simulink model "sf_aero_guidance_fixpt"  (Simulink 6.0)
settings: Solver=ode45  SolverMode=SingleTasking  StartTime=0.0  StopTime=20  RelTol=1e-3  AbsTol=1e-6
PreLoadFcn:
  | aero_guid_dat
InitFcn:
  | ;
StartFcn:
  | ;
StopFcn:
  | aero_guid_plot;
values from neighbouring files (symbols this model uses):
  g = [0.001016 0.001016 0.001016 0.001016 0.001016 0.001016 0.001016 0.001016 0.0010159999994 0.0010159999994 0.0010159999994 0.0010159999994 ... (38 elements, 38x1)]    [sf_electrohydraulic.mat]
  Ks = 8998.87514061    [sf_electrohydraulic.mat]
undefined symbols (not defined in the file or in its folder): Beamwidth, Cm_el, Cm_q, Cz_el, d2r, d_ref, fin_max, fin_min, h_ini, K_r, l_acc, max_acc, max_gimbal, min_gimbal, pos_tgt, S_ref, theta_tgt, Thrust, tors, v_tgt, wgyro, wn_hom, x_ini
libraries: simulink x11, aerospace x5, fixpt_lib_4 x3
Description:
  | The model represents the dynamics of a missile engaging a target which is flying straight and level.
PreSaveFcn:
  | ;
CloseFcn:
  | h=findobj('type','figure');if ~isempty(h);close(h);end;
settings Model: CovMetricSettings=dcmtr  Creator=The MathWorks Inc.  LastModifiedBy=batserve  ExtModeTrigMode=oneshot  ExtModeArmWhenConnect=off  ExtModeAutoUpdateStatusClock=off  ProdHWDeviceType=Specified
settings DataIOCC: LimitDataPoints=off  SaveOutput=off  StateSaveName=xbase  OutputSaveName=ybase  SignalLoggingName=sigsOut
settings OptimizationCC: BlockReduction=off  BooleanDataType=off
settings DebuggingCC: CheckExecutionContextPreStartOutputMsg=on  CheckExecutionContextRuntimeOutputMsg=on  SolverPrmCheckMsg=none  IntegerOverflowMsg=error  ParameterPrecisionLossMsg=none
settings HardwareCC: ProdBitPerShort=32  ProdBitPerInt=16  ProdHWDeviceType=Specified  TargetUnknown=on

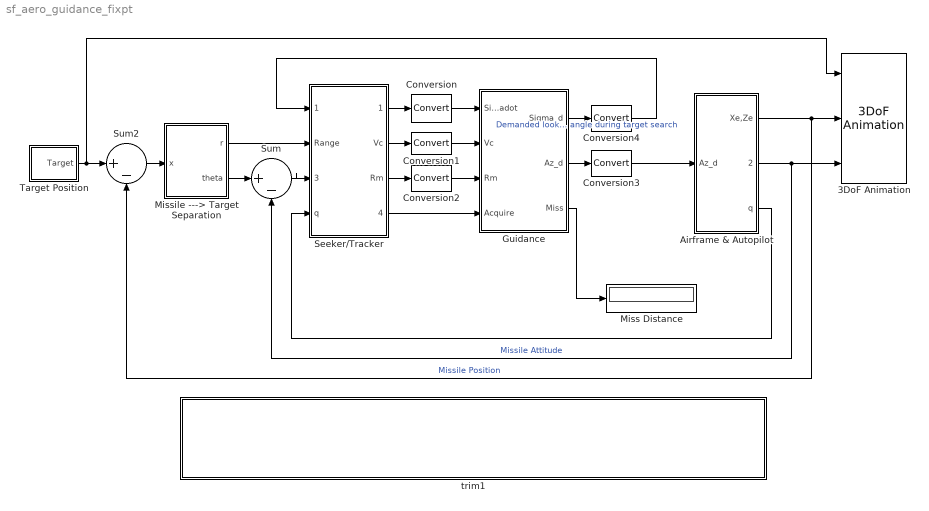
== system sf_aero_guidance_fixpt ==
  3DoF Animation : aerospace/Animation/3DoF Animation  u1=[0 5000 -2000 2000 -5050 -3050]  u2=0.03  u3=1.8  u5=Fly alongside  u6=[200 200 -50]  u7=20  u8=on
  Airframe & Autopilot : Subsystem  PropExecContextAcrossSSBoundary=on
  Conversion : DataTypeConversion  OutDataTypeMode=Specify via dialog  OutScaling=2^-14
  Conversion1 : DataTypeConversion  OutDataTypeMode=Specify via dialog
  Conversion2 : DataTypeConversion  OutScaling=2^-10
  Conversion3 : DataTypeConversion  OutDataTypeMode=Specify via dialog  OutDataType=float('double')  OutScaling=2^-10
  Conversion4 : DataTypeConversion  OutDataTypeMode=Specify via dialog  OutDataType=float('double')  OutScaling=2^-10
  Guidance : Subsystem  PropExecContextAcrossSSBoundary=on
  Miss Distance : Display
  Missile ---> Target Separation : Subsystem  PropExecContextAcrossSSBoundary=on
      mask Type: Cart2Polar
      mask Description:
      | Transformation from cartesian to polar coordinates.
      | [x, y] -> [r, theta]
      | 
      | r = sqrt(x^2 + y^2);
      | theta = atan(y/x);
      mask Help: Unmask this block for more help.
      mask Display: plot(0,0,100,100,[24,20,15,20,20],[85,95,85,95,20],[80,20,95,85,95,85],[70,20,20,15,20,24],[56,56,55,52,50,46],[20,26,31,35,38,42])
  Seeker/Tracker : Subsystem  PropExecContextAcrossSSBoundary=on
  Sum : Sum  Inputs=|+-  SaturateOnIntegerOverflow=on  InputSameDT=on
  Sum2 : Sum  Inputs=|+-  SaturateOnIntegerOverflow=on  InputSameDT=on
  Target Position : Subsystem  PropExecContextAcrossSSBoundary=on
  trim1 : Subsystem  PropExecContextAcrossSSBoundary=on
      settings: AttributesFormatString=\n  OpenFcn=aero_guidance
      mask Display: disp('This model simulates an infrared guidance system using fixed-point math.\n Double-click on this block for the original floating-point version and further details.')
  wires:
  Missile ---> Target Separation/2(theta) -> Sum/1
  Guidance/2(Az_d) -> Conversion3/1
  Seeker/Tracker/2(Vc) -> Conversion1/1
  Seeker/Tracker/3(Rm) -> Conversion2/1
  Guidance/3(Miss) -> Miss Distance/1
  Seeker/Tracker/1(Sigmadot) -> Conversion/1
  Sum/1 -> Seeker/Tracker/3(Look Angle)
  Airframe & Autopilot/3(q) -> Seeker/Tracker/4(q)
  Guidance/1(Sigma_d) -> Conversion4/1  "Demanded look angle during target search"
  Missile ---> Target Separation/1(r) -> Seeker/Tracker/2(Range)
  Airframe & Autopilot/1(Xe,Ze) -> 3DoF Animation/2, Sum2/2  "Missile Position"
  Airframe & Autopilot/2(Attitude) -> 3DoF Animation/3, Sum/2  "Missile Attitude"
  Target Position/1(Target) -> Sum2/1, 3DoF Animation/1
  Sum2/1 -> Missile ---> Target Separation/1(x)
  Seeker/Tracker/4(Acquire) -> Guidance/4(Acquire)
  Conversion/1 -> Guidance/1(Sigmadot)
  Conversion1/1 -> Guidance/2(Vc)
  Conversion2/1 -> Guidance/3(Rm)
  Conversion3/1 -> Airframe & Autopilot/1(Az_d)
  Conversion4/1 -> Seeker/Tracker/1(Sigma_d)

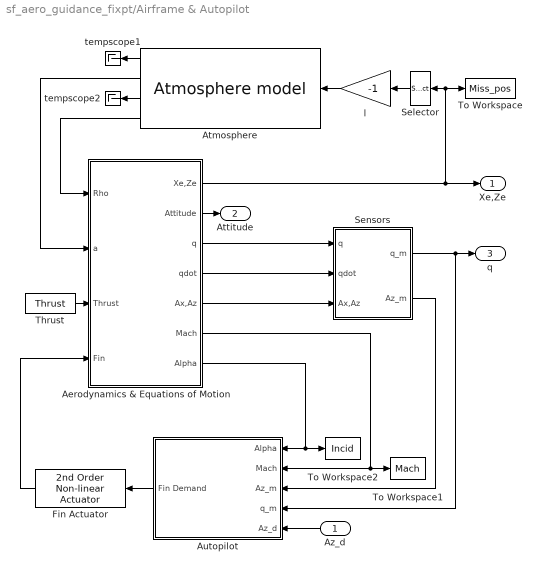
== system sf_aero_guidance_fixpt/Airframe & Autopilot ==
  Az_d : Inport  Orientation=left  Port=1  SampleTime=0  LatchInput=off
  Aerodynamics & Equations of Motion : Subsystem  PropExecContextAcrossSSBoundary=on
  Atmosphere : aerospace/Atmosphere/Atmosphere model  Orientation=left
  Autopilot : Subsystem  Orientation=left  PropExecContextAcrossSSBoundary=on
  Fin Actuator : aerospace/Actuators/2nd Order Non-linear Actuator  Orientation=left  wn_fin=wn_fin  z_fin=z_fin  fin_max=fin_max  fin_min=fin_min  fin_maxrate=fin_maxrate  fin_act_0=fin_act_0
  Selector : Selector  Orientation=left  Elements=[2]  InputPortWidth=2
  Sensors : Subsystem  PropExecContextAcrossSSBoundary=on
  Thrust : Constant  Value=Thrust
  To Workspace : ToWorkspace  VariableName=Miss_pos  SampleTime=-1  SaveFormat=Structure With Time
  To Workspace1 : ToWorkspace  VariableName=Mach  SampleTime=-1  SaveFormat=Structure With Time
  To Workspace2 : ToWorkspace  VariableName=Incid  SampleTime=-1  SaveFormat=Structure With Time
  l : Gain  Orientation=left  Gain=-1  SaturateOnIntegerOverflow=on
  tempscope1 : Terminator
  tempscope2 : Terminator
  Xe,Ze : Outport  InitialOutput=0
  Attitude : Outport  Port=2  InitialOutput=0
  q : Outport  Port=3  InitialOutput=0
  wires:
  Aerodynamics & Equations of Motion/2(Attitude) -> Attitude/1
  Thrust/1 -> Aerodynamics & Equations of Motion/3(Thrust)
  Atmosphere/3 -> tempscope2/1
  Atmosphere/4 -> Aerodynamics & Equations of Motion/1(Rho)
  Atmosphere/1 -> tempscope1/1
  Atmosphere/2 -> Aerodynamics & Equations of Motion/2(a)
  Selector/1 -> l/1
  l/1 -> Atmosphere/1
  Aerodynamics & Equations of Motion/5(Ax,Az) -> Sensors/3(Ax,Az)
  Aerodynamics & Equations of Motion/4(qdot) -> Sensors/2(qdot)
  Aerodynamics & Equations of Motion/1(Xe,Ze) -> Xe,Ze/1, To Workspace/1, Selector/1
  Az_d/1 -> Autopilot/5(Az_d)
  Autopilot/1(Fin Demand) -> Fin Actuator/1
  Fin Actuator/1 -> Aerodynamics & Equations of Motion/4(Fin)
  Aerodynamics & Equations of Motion/7(Alpha) -> Autopilot/1(Alpha), To Workspace2/1
  Sensors/2(Az_m) -> Autopilot/3(Az_m)
  Aerodynamics & Equations of Motion/6(Mach) -> Autopilot/2(Mach), To Workspace1/1
  Sensors/1(q_m) -> Autopilot/4(q_m), q/1
  Aerodynamics & Equations of Motion/3(q) -> Sensors/1(q)

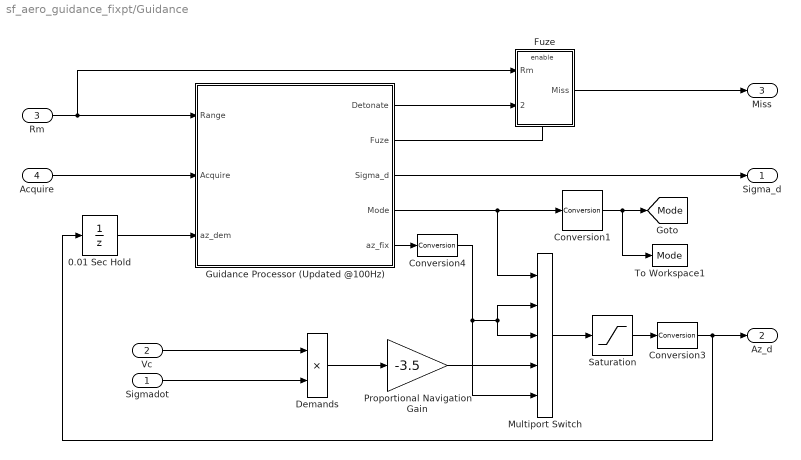
== system sf_aero_guidance_fixpt/Guidance ==
  Sigmadot : Inport  Port=1  SampleTime=0.01  LatchInput=off
  Vc : Inport  Port=2  SampleTime=0.01  LatchInput=off
  Rm : Inport  Port=3  SampleTime=0.01  LatchInput=off
  Acquire : Inport  Port=4  SampleTime=0.01  LatchInput=off
  0.01 Sec Hold : UnitDelay  SampleTime=0.01
  Conversion1 : fixpt_lib_4/Data Type/Conversion  ConvertRealWorld=Real World Value  OutputDataTypeScalingMode=Specify via dialog  OutDataType=float('double')  OutScaling=2^-10  DoSatur=off
  Conversion3 : fixpt_lib_4/Data Type/Conversion  ConvertRealWorld=Real World Value  OutDataType=float('double')  OutScaling=2^-10  DoSatur=off
  Conversion4 : fixpt_lib_4/Data Type/Conversion  ConvertRealWorld=Real World Value  OutDataType=float('double')  OutScaling=2^-10  DoSatur=off
  Demands : Product  OutDataTypeMode=Specify via dialog  OutScaling=2^-6  SaturateOnIntegerOverflow=on
  Fuze : Subsystem  TreatAsAtomicUnit=on  PropExecContextAcrossSSBoundary=on
  Guidance Processor (Updated @100Hz) : Stateflow chart  PropExecContextAcrossSSBoundary=on
  Multiport Switch : MultiPortSwitch  InputSameDT=on
  Proportional Navigation Gain : Gain  Gain=-3.5  SaturateOnIntegerOverflow=on
  Saturation : Saturate  UpperLimit=max_acc  LowerLimit=-max_acc
  To Workspace1 : ToWorkspace  VariableName=Mode  SaveFormat=Structure With Time
  Sigma_d : Outport
  Az_d : Outport  Port=2
  Miss : Outport  Port=3
  tag scope: Mode=global
  wires:
  Fuze/1("Miss ") -> Miss/1
  Rm/1 -> Guidance Processor (Updated @100Hz)/1(Range), Fuze/1(Rm)
  Guidance Processor (Updated @100Hz)/4(Mode) -> Multiport Switch/1, Conversion1/1
  Acquire/1 -> Guidance Processor (Updated @100Hz)/2(Acquire)
  Multiport Switch/1 -> Saturation/1
  Saturation/1 -> Conversion3/1
  Guidance Processor (Updated @100Hz)/5(az_fix) -> Conversion4/1
  0.01 Sec Hold/1 -> Guidance Processor (Updated @100Hz)/3(az_dem)
  Guidance Processor (Updated @100Hz)/2(Fuze) -> Fuze/Enable
  Sigmadot/1 -> Demands/2
  Proportional Navigation Gain/1 -> Multiport Switch/4
  Vc/1 -> Demands/1
  Demands/1 -> Proportional Navigation Gain/1
  Guidance Processor (Updated @100Hz)/3(Sigma_d) -> Sigma_d/1
  Conversion1/1 -> [Mode], To Workspace1/1
  Guidance Processor (Updated @100Hz)/1(Detonate) -> Fuze/2(Detonate)
  Conversion3/1 -> Az_d/1, 0.01 Sec Hold/1
  Conversion4/1 -> Multiport Switch/2, Multiport Switch/3, Multiport Switch/5

== system sf_aero_guidance_fixpt/Missile ---> Target Separation ==
  x : Inport  Port=1  LatchInput=off
  Range : Fcn  Expr=hypot(u[1],u[2])
  Sightline Angle : Fcn  Expr=atan2(-u[2],u[1])
  r : Outport  InitialOutput=0
  theta : Outport  Port=2  InitialOutput=0
  wires:
  x/1 -> Sightline Angle/1, Range/1
  Range/1 -> r/1
  Sightline Angle/1 -> theta/1

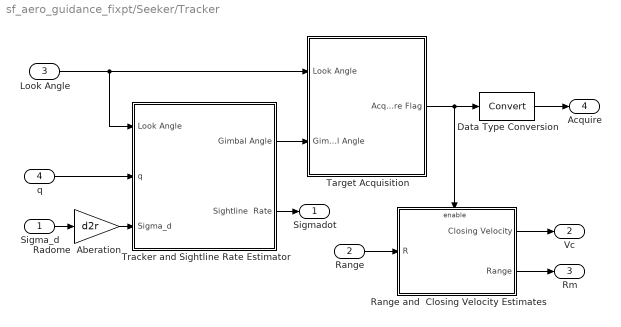
== system sf_aero_guidance_fixpt/Seeker/Tracker ==
  Sigma_d : Inport  Port=1  LatchInput=off
  Range : Inport  Port=2  LatchInput=off
  Look Angle : Inport  Port=3  LatchInput=off
  q : Inport  Port=4  LatchInput=off
  Data Type Conversion : DataTypeConversion  OutDataTypeMode=boolean  SaturateOnIntegerOverflow=on  RndMeth=Zero
  Radome  Aberation : Gain  Gain=d2r  SaturateOnIntegerOverflow=on
  Range and  Closing Velocity Estimates : Subsystem  TreatAsAtomicUnit=on  PropExecContextAcrossSSBoundary=on
  Target Acquisition : Subsystem  PropExecContextAcrossSSBoundary=on
  Tracker and Sightline Rate Estimator : Subsystem  PropExecContextAcrossSSBoundary=on
  Sigmadot : Outport
  Vc : Outport  Port=2
  Rm : Outport  Port=3
  Acquire : Outport  Port=4
  wires:
  Tracker and Sightline Rate Estimator/2(Sightline  Rate) -> Sigmadot/1
  Radome  Aberation/1 -> Tracker and Sightline Rate Estimator/3(Sigma_d)
  Tracker and Sightline Rate Estimator/1("Gimbal Angle ") -> Target Acquisition/2(Gimbal Angle)
  Target Acquisition/1(Acquire Flag) -> Range and  Closing Velocity Estimates/Enable, Data Type Conversion/1
  q/1 -> Tracker and Sightline Rate Estimator/2(q)
  Look Angle/1 -> Target Acquisition/1(Look Angle), Tracker and Sightline Rate Estimator/1(Look Angle)
  Range/1 -> Range and  Closing Velocity Estimates/1(R)
  Range and  Closing Velocity Estimates/2(Range) -> Rm/1
  Range and  Closing Velocity Estimates/1(Closing Velocity) -> Vc/1
  Sigma_d/1 -> Radome  Aberation/1
  Data Type Conversion/1 -> Acquire/1

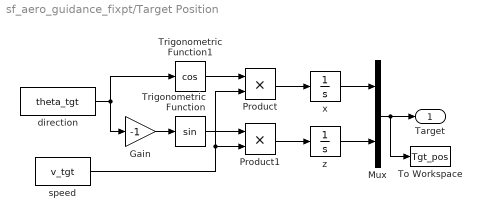
== system sf_aero_guidance_fixpt/Target Position ==
  Gain : Gain  Gain=-1  SaturateOnIntegerOverflow=on
  Mux : Mux  Inputs=2
  Product : Product  SaturateOnIntegerOverflow=on  InputSameDT=on
  Product1 : Product  SaturateOnIntegerOverflow=on  InputSameDT=on
  To Workspace : ToWorkspace  VariableName=Tgt_pos  SampleTime=-1  SaveFormat=Structure
  Trigonometric Function : Trigonometry
  Trigonometric Function1 : Trigonometry  Operator=cos
  direction : Constant  Value=theta_tgt
  speed : Constant  Value=v_tgt
  x : Integrator  InitialCondition=pos_tgt(1)  ZeroCross=off
  z : Integrator  InitialCondition=pos_tgt(2)  ZeroCross=off
  Target : Outport
  wires:
  x/1 -> Mux/1
  z/1 -> Mux/2
  Product/1 -> x/1
  Product1/1 -> z/1
  speed/1 -> Product/2, Product1/2
  Trigonometric Function/1 -> Product1/1
  Trigonometric Function1/1 -> Product/1
  direction/1 -> Trigonometric Function1/1, Gain/1
  Gain/1 -> Trigonometric Function/1
  Mux/1 -> Target/1, To Workspace/1

== system sf_aero_guidance_fixpt/trim1 ==

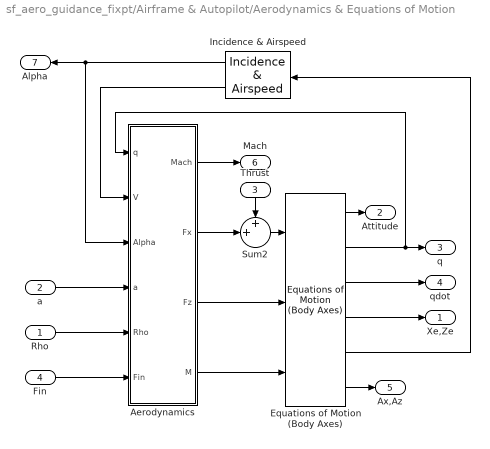
== system sf_aero_guidance_fixpt/Airframe & Autopilot/Aerodynamics & Equations of Motion ==
  Rho : Inport  Port=1  LatchInput=off
  a : Inport  Port=2  LatchInput=off
  Thrust : Inport  Orientation=down  Port=3  LatchInput=off
  Fin : Inport  Port=4  LatchInput=off
  " Equations of Motion (Body Axes)" : aerospace/3DoF Equations of Motion / Equations of Motion (Body Axes)  v_ini=v_ini  theta_ini=theta_ini  alpha_ini=alpha_ini  q_ini=q_ini  pos_ini=[x_ini -h_ini]  mass=mass  Iyy=Iyy  g=g
  Aerodynamics : Subsystem  PropExecContextAcrossSSBoundary=on
  Incidence & Airspeed : aerospace/3DoF Equations of Motion /Incidence  & Airspeed  Orientation=left
  Sum2 : Sum  Inputs=++|  SaturateOnIntegerOverflow=on  InputSameDT=on
  Xe,Ze : Outport  InitialOutput=0
  Attitude : Outport  Port=2  InitialOutput=0
  q : Outport  Port=3  InitialOutput=0
  qdot : Outport  Port=4  InitialOutput=0
  Ax,Az : Outport  Port=5  InitialOutput=0
  Mach : Outport  Port=6  InitialOutput=0
  Alpha : Outport  Orientation=left  Port=7  InitialOutput=0
  wires:
  Aerodynamics/1(" Mach") -> Mach/1
  Aerodynamics/4(" M") -> " Equations of Motion (Body Axes)"/3
  Sum2/1 -> " Equations of Motion (Body Axes)"/1
  Incidence & Airspeed/1 -> Aerodynamics/3(Alpha), Alpha/1
  Rho/1 -> Aerodynamics/5(Rho)
  a/1 -> Aerodynamics/4(a)
  Fin/1 -> Aerodynamics/6(Fin)
  Incidence & Airspeed/2 -> Aerodynamics/2(V)
  Aerodynamics/3(Fz) -> " Equations of Motion (Body Axes)"/2
  Aerodynamics/2(Fx) -> Sum2/2
  Thrust/1 -> Sum2/1
  " Equations of Motion (Body Axes)"/2 -> q/1, Aerodynamics/1(q)
  " Equations of Motion (Body Axes)"/3 -> qdot/1
  " Equations of Motion (Body Axes)"/1 -> Attitude/1
  " Equations of Motion (Body Axes)"/4 -> Xe,Ze/1
  " Equations of Motion (Body Axes)"/6 -> Ax,Az/1
  " Equations of Motion (Body Axes)"/5 -> Incidence & Airspeed/1

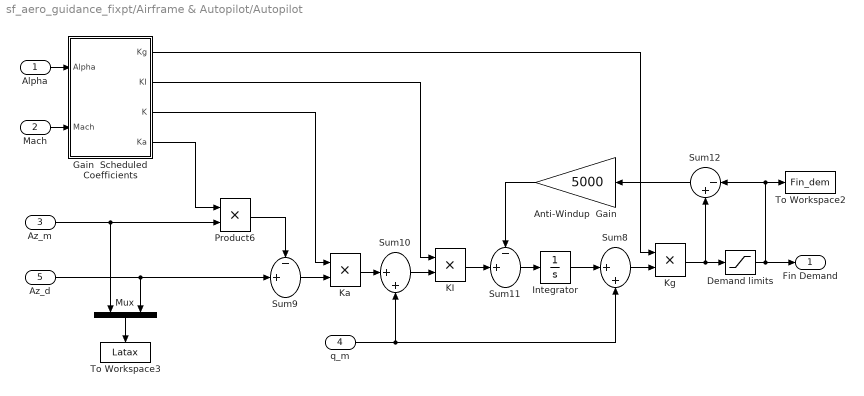
== system sf_aero_guidance_fixpt/Airframe & Autopilot/Autopilot ==
  Alpha : Inport  Port=1  LatchInput=off
  Mach : Inport  Port=2  LatchInput=off
  Az_m : Inport  Port=3  LatchInput=off
  q_m : Inport  Port=4  LatchInput=off
  Az_d : Inport  Port=5  LatchInput=off
  Anti-Windup  Gain : Gain  Orientation=left  Gain=5000  SaturateOnIntegerOverflow=on
  "Demand limits " : Saturate  UpperLimit=fin_max  LowerLimit=fin_min  ZeroCross=off
  Gain  Scheduled Coefficients : Subsystem  PropExecContextAcrossSSBoundary=on
  Integrator : Integrator  ZeroCross=off
  KI : Product  SaturateOnIntegerOverflow=on  InputSameDT=on
  Ka : Product  SaturateOnIntegerOverflow=on  InputSameDT=on
  Kg : Product  SaturateOnIntegerOverflow=on  InputSameDT=on
  Mux : Mux  Orientation=down  Inputs=2
  Product6 : Product  SaturateOnIntegerOverflow=on  InputSameDT=on
  Sum10 : Sum  Inputs=|++  SaturateOnIntegerOverflow=on  InputSameDT=on
  Sum11 : Sum  Inputs=-+|  SaturateOnIntegerOverflow=on  InputSameDT=on
  Sum12 : Sum  Orientation=left  Inputs=|-+  SaturateOnIntegerOverflow=on  InputSameDT=on
  Sum8 : Sum  Inputs=|++  SaturateOnIntegerOverflow=on  InputSameDT=on
  Sum9 : Sum  Inputs=-+|  SaturateOnIntegerOverflow=on  InputSameDT=on
  To Workspace2 : ToWorkspace  VariableName=Fin_dem  SampleTime=-1  SaveFormat=Structure With Time
  To Workspace3 : ToWorkspace  VariableName=Latax  SampleTime=-1  SaveFormat=Structure With Time
      settings: Orientation=down
  Fin Demand : Outport  InitialOutput=0
  wires:
  Mach/1 -> Gain  Scheduled Coefficients/2(Mach)
  Alpha/1 -> Gain  Scheduled Coefficients/1(Alpha)
  Kg/1 -> Sum12/2, "Demand limits "/1
  Gain  Scheduled Coefficients/1("Kg ") -> Kg/1
  Gain  Scheduled Coefficients/3("K ") -> Ka/1
  Gain  Scheduled Coefficients/2("KI ") -> KI/1
  Anti-Windup  Gain/1 -> Sum11/1
  Sum8/1 -> Kg/2
  Integrator/1 -> Sum8/1
  Sum11/1 -> Integrator/1
  Product6/1 -> Sum9/1
  Sum9/1 -> Ka/2
  Ka/1 -> Sum10/1
  Sum10/1 -> KI/2
  KI/1 -> Sum11/2
  Sum12/1 -> Anti-Windup  Gain/1
  Az_d/1 -> Mux/2, Sum9/2
  Mux/1 -> To Workspace3/1
  q_m/1 -> Sum10/2, Sum8/2
  "Demand limits "/1 -> Fin Demand/1, Sum12/1, To Workspace2/1
  Az_m/1 -> Mux/1, Product6/2
  Gain  Scheduled Coefficients/4("Ka ") -> Product6/1

== system sf_aero_guidance_fixpt/Airframe & Autopilot/Sensors ==
  q : Inport  Port=1  LatchInput=off
  qdot : Inport  Port=2  LatchInput=off
  Ax,Az : Inport  Port=3  LatchInput=off
  Selector : Selector  Elements=[2]  InputPortWidth=2
  Sum : Sum  Inputs=-+|  SaturateOnIntegerOverflow=on  InputSameDT=on
  l : Gain  Gain=l_acc  SaturateOnIntegerOverflow=on
  q_m : Outport  InitialOutput=0
  Az_m : Outport  Port=2  InitialOutput=0
  wires:
  Selector/1 -> Sum/2
  Ax,Az/1 -> Selector/1
  q/1 -> q_m/1  "Rate Gyro"
  l/1 -> Sum/1
  Sum/1 -> Az_m/1  "Accelerometer"
  qdot/1 -> l/1

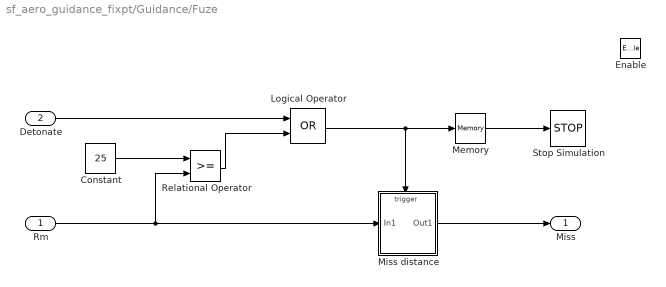
== system sf_aero_guidance_fixpt/Guidance/Fuze ==
  Rm : Inport  Port=1  LatchInput=off
  Detonate : Inport  Port=2  LatchInput=off
  Enable : EnablePort  ZeroCross=off
  Constant : Constant  Value=25
  Logical Operator : Logic  Operator=OR
  Memory : Memory  InheritSampleTime=on
  Miss distance : Subsystem  TreatAsAtomicUnit=on  PropExecContextAcrossSSBoundary=on
  Relational Operator : RelationalOperator  LogicOutDataTypeMode=Boolean
  Stop Simulation : Stop
  "Miss " : Outport
  wires:
  Detonate/1 -> Logical Operator/1
  Rm/1 -> Miss distance/1(In1), Relational Operator/2
  Relational Operator/1 -> Logical Operator/2
  Memory/1 -> Stop Simulation/1
  Miss distance/1(Out1) -> "Miss "/1
  Logical Operator/1 -> Miss distance/Trigger, Memory/1
  Constant/1 -> Relational Operator/1

== system sf_aero_guidance_fixpt/Seeker/Tracker/Range and  Closing Velocity Estimates ==
  R : Inport  Port=1  LatchInput=off
  Enable : EnablePort  Orientation=left  StatesWhenEnabling=reset  ZeroCross=off
  Bandwidth of Estimator : Gain  Gain=wn_hom  SaturateOnIntegerOverflow=on
  Initialized at acquisition : Integrator  Orientation=left  InitialConditionSource=external  ZeroCross=off
  Rdot ---> Vc : Gain  Gain=-1  SaturateOnIntegerOverflow=on
  Sum : Sum  Inputs=|+-  SaturateOnIntegerOverflow=on  InputSameDT=on
  Closing Velocity : Outport  InitialOutput=0
  Range : Outport  Port=2  InitialOutput=0
  wires:
  R/1 -> Range/1, Initialized at acquisition/2, Sum/1
  Sum/1 -> Bandwidth of Estimator/1
  Initialized at acquisition/1 -> Sum/2
  Bandwidth of Estimator/1 -> Rdot ---> Vc/1, Initialized at acquisition/1
  Rdot ---> Vc/1 -> Closing Velocity/1

== system sf_aero_guidance_fixpt/Seeker/Tracker/Target Acquisition ==
  Look Angle : Inport  Port=1  LatchInput=off
  Gimbal Angle : Inport  Port=2  LatchInput=off
  Abs : Abs  SaturateOnIntegerOverflow=on
  Beamwidth : Constant  Value=Beamwidth/2
  Mux : Mux  Inputs=2
  Relational Operator : RelationalOperator  Operator=<  InputSameDT=on
  Sum : Sum  Inputs=+-  SaturateOnIntegerOverflow=on  InputSameDT=on
  To Workspace2 : ToWorkspace  VariableName=Gimbal  SampleTime=-1  SaveFormat=Structure With Time
  Acquire Flag : Outport
  wires:
  Look Angle/1 -> Sum/2, Mux/2
  Gimbal Angle/1 -> Sum/1, Mux/1
  Mux/1 -> To Workspace2/1
  Sum/1 -> Abs/1
  Beamwidth/1 -> Relational Operator/2
  Relational Operator/1 -> Acquire Flag/1
  Abs/1 -> Relational Operator/1

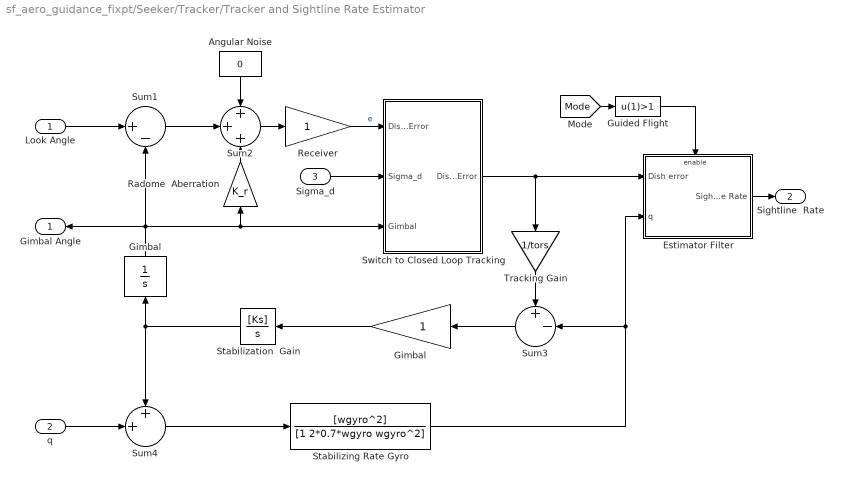
== system sf_aero_guidance_fixpt/Seeker/Tracker/Tracker and Sightline Rate Estimator ==
  Look Angle : Inport  Port=1  LatchInput=off
  q : Inport  Port=2  LatchInput=off
  Sigma_d : Inport  Port=3  LatchInput=off
  Angular Noise : Constant  Orientation=down  Value=0
  Estimator Filter : Subsystem  TreatAsAtomicUnit=on  PropExecContextAcrossSSBoundary=on
  Gimbal : Gain  Orientation=left  SaturateOnIntegerOverflow=on
  "Gimbal " : Integrator  Orientation=up  LimitOutput=on  UpperSaturationLimit=max_gimbal  LowerSaturationLimit=min_gimbal  ZeroCross=off
  Guided Flight : Fcn  Expr=u(1)>1
  Radome  Aberration : Gain  Orientation=up  Gain=K_r  SaturateOnIntegerOverflow=on
  Receiver : Gain  SaturateOnIntegerOverflow=on
  Stabilization  Gain : TransferFcn  Orientation=left  Numerator=[Ks]  Denominator=[1 0]
  Stabilizing Rate Gyro : TransferFcn  Numerator=[wgyro^2]  Denominator=[1 2*0.7*wgyro wgyro^2]
  Sum1 : Sum  Inputs=|+-  SaturateOnIntegerOverflow=on  InputSameDT=on
  Sum2 : Sum  Inputs=+++  SaturateOnIntegerOverflow=on  InputSameDT=on
  Sum3 : Sum  Orientation=left  Inputs=+-|  SaturateOnIntegerOverflow=on  InputSameDT=on
  Sum4 : Sum  Inputs=++|  SaturateOnIntegerOverflow=on  InputSameDT=on
  Switch to Closed Loop Tracking : Subsystem  PropExecContextAcrossSSBoundary=on
  Tracking Gain : Gain  Orientation=down  Gain=1/tors  SaturateOnIntegerOverflow=on
  "Gimbal Angle " : Outport  Orientation=left
  Sightline  Rate : Outport  Port=2
  wires:
  "Gimbal "/1 -> Sum1/2, Radome  Aberration/1, Switch to Closed Loop Tracking/3(Gimbal), "Gimbal Angle "/1
  Stabilization  Gain/1 -> "Gimbal "/1, Sum4/1
  Gimbal/1 -> Stabilization  Gain/1
  Look Angle/1 -> Sum1/1
  Sum2/1 -> Receiver/1
  Receiver/1 -> Switch to Closed Loop Tracking/1(Dish Error)  "e"
  Sigma_d/1 -> Switch to Closed Loop Tracking/2(Sigma_d)
  Estimator Filter/1(Sightline Rate) -> Sightline  Rate/1
  Radome  Aberration/1 -> Sum2/3
  Sum1/1 -> Sum2/2
  Angular Noise/1 -> Sum2/1
  Sum4/1 -> Stabilizing Rate Gyro/1
  q/1 -> Sum4/2
  Stabilizing Rate Gyro/1 -> Sum3/2, Estimator Filter/2(q)
  Sum3/1 -> Gimbal/1
  Tracking Gain/1 -> Sum3/1
  Switch to Closed Loop Tracking/1(Dish Error) -> Tracking Gain/1, Estimator Filter/1(Dish error)
  Guided Flight/1 -> Estimator Filter/Enable
  [Mode] -> Guided Flight/1

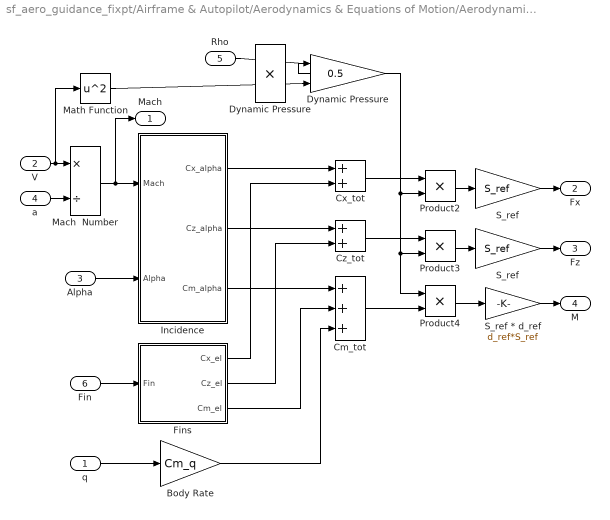
== system sf_aero_guidance_fixpt/Airframe & Autopilot/Aerodynamics & Equations of Motion/Aerodynamics ==
  q : Inport  Port=1  LatchInput=off
  V : Inport  Port=2  LatchInput=off
  Alpha : Inport  Port=3  LatchInput=off
  a : Inport  Port=4  LatchInput=off
  Rho : Inport  Port=5  LatchInput=off
  Fin : Inport  Port=6  LatchInput=off
  Body Rate : Gain  Gain=Cm_q  SaturateOnIntegerOverflow=on
  Cm_tot : Sum  Inputs=+++  SaturateOnIntegerOverflow=on  InputSameDT=on
  Cx_tot : Sum  SaturateOnIntegerOverflow=on  InputSameDT=on
  Cz_tot : Sum  SaturateOnIntegerOverflow=on  InputSameDT=on
  Dynamic Pressure : Gain  Gain=0.5  SaturateOnIntegerOverflow=on
  Dynamic Pressure : Product  SaturateOnIntegerOverflow=on  InputSameDT=on
  Fins : Subsystem  PropExecContextAcrossSSBoundary=on
  Incidence : Subsystem  PropExecContextAcrossSSBoundary=on
  Mach  Number : Product  Inputs=*/  SaturateOnIntegerOverflow=on  InputSameDT=on
  Math Function : Math  Operator=square  SaturateOnIntegerOverflow=on
  Product2 : Product  SaturateOnIntegerOverflow=on  InputSameDT=on
  Product3 : Product  SaturateOnIntegerOverflow=on  InputSameDT=on
  Product4 : Product  SaturateOnIntegerOverflow=on  InputSameDT=on
  S_ref : Gain  Gain=S_ref  SaturateOnIntegerOverflow=on
  S_ref * d_ref : Gain  Gain=d_ref*S_ref  SaturateOnIntegerOverflow=on
  "S_ref " : Gain  Gain=S_ref  SaturateOnIntegerOverflow=on
  " Mach" : Outport  InitialOutput=0
  Fx : Outport  Port=2  InitialOutput=[0]
  Fz : Outport  Port=3  InitialOutput=0
  " M" : Outport  Port=4  InitialOutput=0
  wires:
  Math Function/1 -> Dynamic Pressure/2
  Rho/1 -> Dynamic Pressure/1
  Dynamic Pressure/1 -> Dynamic Pressure/1
  Dynamic Pressure/1 -> Product2/2, Product3/2, Product4/1
  V/1 -> Math Function/1, Mach  Number/1
  Incidence/1(Cx_alpha) -> Cx_tot/1
  Fins/1(Cx_el) -> Cx_tot/2
  Incidence/2(Cz_alpha) -> Cz_tot/1
  Fins/2(Cz_el) -> Cz_tot/2
  Incidence/3(Cm_alpha) -> Cm_tot/1
  Fins/3(Cm_el) -> Cm_tot/2
  Body Rate/1 -> Cm_tot/3
  a/1 -> Mach  Number/2
  Alpha/1 -> Incidence/2(Alpha)
  Cx_tot/1 -> Product2/1
  Cz_tot/1 -> Product3/1
  Product2/1 -> S_ref/1
  S_ref/1 -> Fx/1
  Product3/1 -> "S_ref "/1
  "S_ref "/1 -> Fz/1
  Fin/1 -> Fins/1(Fin)
  S_ref * d_ref/1 -> " M"/1
  Product4/1 -> S_ref * d_ref/1
  Cm_tot/1 -> Product4/2
  q/1 -> Body Rate/1
  Mach  Number/1 -> " Mach"/1, Incidence/1(Mach)

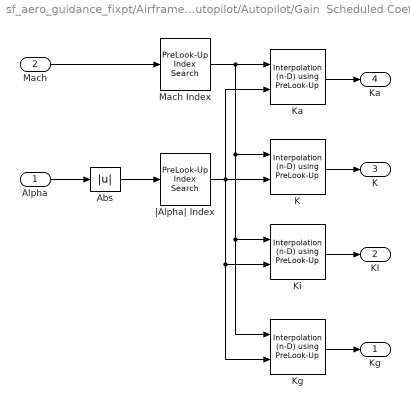
== system sf_aero_guidance_fixpt/Airframe & Autopilot/Autopilot/Gain  Scheduled Coefficients ==
  Alpha : Inport  Port=1  LatchInput=off
  Mach : Inport  Port=2  LatchInput=off
  Abs : Abs  SaturateOnIntegerOverflow=on
  K : simulink/Look-Up Tables/Interpolation (n-D) using PreLook-Up  numDimsPopupSelect=2  explicitNumDims=2  table=K  interpMethod=Linear  extrapMethod=Linear  rangeErrorMode=None
  Ka : simulink/Look-Up Tables/Interpolation (n-D) using PreLook-Up  numDimsPopupSelect=2  explicitNumDims=2  table=Ka  interpMethod=Linear  extrapMethod=Linear  rangeErrorMode=None
  Kg : simulink/Look-Up Tables/Interpolation (n-D) using PreLook-Up  numDimsPopupSelect=2  explicitNumDims=2  table=Kg  interpMethod=Linear  extrapMethod=Linear  rangeErrorMode=None
  Ki : simulink/Look-Up Tables/Interpolation (n-D) using PreLook-Up  numDimsPopupSelect=2  explicitNumDims=2  table=Ki  interpMethod=Linear  extrapMethod=Linear  rangeErrorMode=None
  Mach Index : simulink/Look-Up Tables/PreLook-Up Index Search  bpData=M_sch  searchMode=Binary Search  cacheBpFlag=on  outputFlag=off  extrapMode=Linear Extrapolation  rangeErrorMode=None
  |Alpha| Index : simulink/Look-Up Tables/PreLook-Up Index Search  bpData=alpha_sch  searchMode=Binary Search  cacheBpFlag=on  outputFlag=off  extrapMode=Linear Extrapolation  rangeErrorMode=None
  "Kg " : Outport  InitialOutput=0
  "KI " : Outport  Port=2  InitialOutput=0
  "K " : Outport  Port=3  InitialOutput=0
  "Ka " : Outport  Port=4  InitialOutput=0
  wires:
  Alpha/1 -> Abs/1
  Mach Index/1 -> Ka/1, K/1, Ki/1, Kg/1
  |Alpha| Index/1 -> Ka/2, K/2, Ki/2, Kg/2
  Ka/1 -> "Ka "/1
  K/1 -> "K "/1
  Ki/1 -> "KI "/1
  Kg/1 -> "Kg "/1
  Abs/1 -> |Alpha| Index/1
  Mach/1 -> Mach Index/1

== system sf_aero_guidance_fixpt/Guidance/Fuze/Miss distance ==
  In1 : Inport  Port=1  LatchInput=off
  Trigger : TriggerPort
  Out1 : Outport
  wires:
  In1/1 -> Out1/1

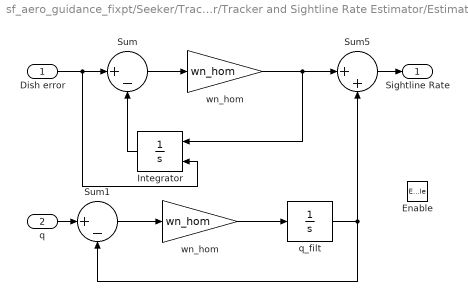
== system sf_aero_guidance_fixpt/Seeker/Tracker/Tracker and Sightline Rate Estimator/Estimator Filter ==
  Dish error : Inport  Port=1  LatchInput=off
  q : Inport  Port=2  LatchInput=off
  Enable : EnablePort  StatesWhenEnabling=reset  ZeroCross=off
  Integrator : Integrator  Orientation=left  InitialConditionSource=external  ZeroCross=off
  Sum : Sum  Inputs=|+-  SaturateOnIntegerOverflow=on  InputSameDT=on
  Sum1 : Sum  Inputs=|+-  SaturateOnIntegerOverflow=on  InputSameDT=on
  Sum5 : Sum  Inputs=|++  SaturateOnIntegerOverflow=on  InputSameDT=on
  q_filt : Integrator  ZeroCross=off
  wn_hom : Gain  Gain=wn_hom  SaturateOnIntegerOverflow=on
  "wn_hom  " : Gain  Gain=wn_hom  SaturateOnIntegerOverflow=on
  Sightline Rate : Outport  InitialOutput=0
  wires:
  Dish error/1 -> Sum/1, Integrator/2
  Sum/1 -> wn_hom/1
  Integrator/1 -> Sum/2
  Sum5/1 -> Sightline Rate/1
  wn_hom/1 -> Integrator/1, Sum5/1
  q/1 -> Sum1/1
  Sum1/1 -> "wn_hom  "/1
  "wn_hom  "/1 -> q_filt/1
  q_filt/1 -> Sum5/2, Sum1/2

== system sf_aero_guidance_fixpt/Seeker/Tracker/Tracker and Sightline Rate Estimator/Switch to Closed Loop Tracking ==
  Dish Error : Inport  Port=1  LatchInput=off
  Sigma_d : Inport  Port=2  LatchInput=off
  Gimbal : Inport  Port=3  LatchInput=off
  Guided Flight : Fcn  Expr=u(1)>1
  Sum5 : Sum  Inputs=-+  SaturateOnIntegerOverflow=on  InputSameDT=on
  Switch2 : Switch  Threshold=0.5  InputSameDT=on
  Dish Error : Outport
  wires:
  [Mode] -> Guided Flight/1
  Guided Flight/1 -> Switch2/2
  Sum5/1 -> Switch2/3
  Dish Error/1 -> Switch2/1
  Switch2/1 -> Dish Error/1
  Sigma_d/1 -> Sum5/2
  Gimbal/1 -> Sum5/1

== system sf_aero_guidance_fixpt/Airframe & Autopilot/Aerodynamics & Equations of Motion/Aerodynamics/Fins ==
  Fin : Inport  Port=1  LatchInput=off
  Cm : Gain  Gain=Cm_el  SaturateOnIntegerOverflow=on
  Cx : Gain  Gain=0  SaturateOnIntegerOverflow=on
  Cz : Gain  Gain=Cz_el  SaturateOnIntegerOverflow=on
  Cx_el : Outport  InitialOutput=0
  Cz_el : Outport  Port=2  InitialOutput=0
  Cm_el : Outport  Port=3  InitialOutput=0
  wires:
  Fin/1 -> Cx/1, Cm/1, Cz/1
  Cx/1 -> Cx_el/1
  Cm/1 -> Cm_el/1
  Cz/1 -> Cz_el/1

== system sf_aero_guidance_fixpt/Airframe & Autopilot/Aerodynamics & Equations of Motion/Aerodynamics/Incidence ==
  Mach : Inport  Port=1  LatchInput=off
  Alpha : Inport  Port=2  LatchInput=off
  Alpha Index : simulink/Look-Up Tables/PreLook-Up Index Search  bpData=alpha_vec  searchMode=Binary Search  cacheBpFlag=on  outputFlag=off  extrapMode=Linear Extrapolation  rangeErrorMode=None
  Cm : simulink/Look-Up Tables/Interpolation (n-D) using PreLook-Up  numDimsPopupSelect=2  explicitNumDims=2  table=Cm_alpha  interpMethod=Linear  extrapMethod=Linear  rangeErrorMode=None
  Cx : simulink/Look-Up Tables/Interpolation (n-D) using PreLook-Up  numDimsPopupSelect=2  explicitNumDims=2  table=Cx_alpha  interpMethod=Linear  extrapMethod=Linear  rangeErrorMode=None
  Cz : simulink/Look-Up Tables/Interpolation (n-D) using PreLook-Up  numDimsPopupSelect=2  explicitNumDims=2  table=Cz_alpha  interpMethod=Linear  extrapMethod=Linear  rangeErrorMode=None
  Mach Index : simulink/Look-Up Tables/PreLook-Up Index Search  bpData=Mach_vec  searchMode=Binary Search  cacheBpFlag=on  outputFlag=off  extrapMode=Linear Extrapolation  rangeErrorMode=None
  Cx_alpha : Outport  InitialOutput=0
  Cz_alpha : Outport  Port=2  InitialOutput=0
  Cm_alpha : Outport  Port=3  InitialOutput=0
  wires:
  Alpha Index/1 -> Cx/1, Cz/1, Cm/1
  Mach Index/1 -> Cx/2, Cz/2, Cm/2
  Cx/1 -> Cx_alpha/1
  Cz/1 -> Cz_alpha/1
  Cm/1 -> Cm_alpha/1
  Alpha/1 -> Alpha Index/1
  Mach/1 -> Mach Index/1

== stateflow chart Guidance/Guidance Processor (Updated @100Hz) ==
  settings: updateMethod=DISCRETE  sampleTime=0.01  executeAtInitialization=1
  state Guidance [parallel]
    state Target_Search
      en: Mode=1;Sigma_d=0;incr=-100;
      du: Sigma_d=Sigma_d+0.01C*incr;
      Target_Search -> Target_Search : [Sigma_d>30||Sigma_d<-30]  / incr=-incr;
    state Target_Lock
      en:Mode=2;
    state Abort
      en:Detonate=1;
    state Radar_Guided
      en:Mode=3;
      ex:az_fix=az_dem;
    state Blind_Range
      en:Mode=4;
    (default) -> Target_Search : {az_fix=-9.81C;}
    Radar_Guided -> Target_Search : [Acquire==0]
    Target_Search -> Abort : after(700,wakeup) / Timeout;
    Target_Search -> Target_Lock : [Acquire==1]
    Target_Lock -> Radar_Guided : after(20,wakeup)
    Radar_Guided -> Blind_Range : [Range<200]
  state Fuze [parallel]
    state Inert
      en:Fuze = 0;
    state Armed
      en:Fuze=1;
    (default) -> Inert
    Armed -> Inert : enter(Guidance.Target_Search)
    Inert -> Armed : Timeout
    Inert -> Armed : [in(Guidance.Radar_Guided)&&Range<1000]
  data: Range input fixpt; Detonate output boolean; Fuze output boolean; Sigma_d output fixpt; Mode output uint8; Acquire input boolean; incr local int16; az_dem input fixpt; az_fix output fixpt =-9.81
  data Range settings: units=metres
  data Sigma_d settings: units=deg  description=Demanded Seeker Look Angle
  data Acquire settings: description=Seeker Acquisition Flag
  data incr settings: units=deg/sec  description=Seeker Search Rate
  events: Timeout local EITHER_EDGE_EVENT
